simulink model "control_sim_PI_non_linear_noise"  (R2024b)
settings: Solver=ode4  StartTime=0.0  StopTime=150  FixedStep=0.001  RelTol=1e-3
libraries: simulink x1, slpidlib x1
settings Model: Creator=henri  LastModifiedBy=guilherme-lazzarini
settings ConfigComp: CovBoundaryAbsTol=1.0e-5

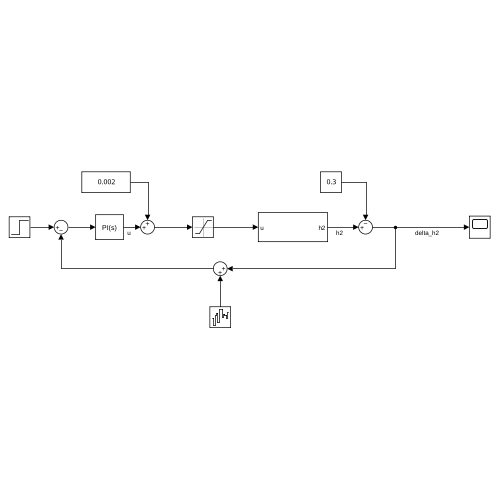
[thumbnail: Simulink's stored preview of the top-level diagram]
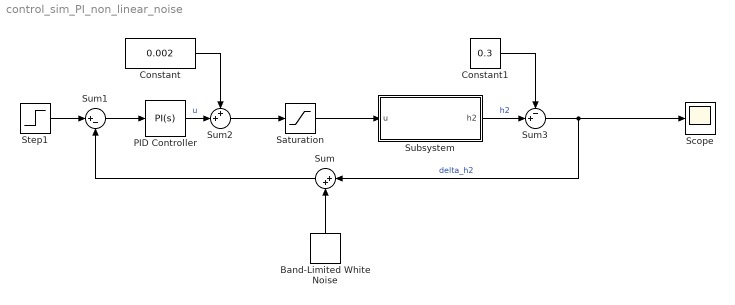
== system control_sim_PI_non_linear_noise ==
  Band-Limited White Noise : simulink/Sources/Band-Limited White Noise  Cov=[0.0001]  Ts=0.1  seed=[23341]
  Constant : Constant  Value=0.002
  Constant1 : Constant  Value=0.3
  PID Controller : slpidlib/PID Controller  Controller=PI  Form=Parallel  TimeDomain=Continuous-time  UseExternalTs=off  SampleTime=-1  IntegratorMethod=Forward Euler  FilterMethod=Forward Euler  ControllerParametersSource=internal  P=0.17  I=0.005  UseKiTs=off  D=1.75  UseExternalDerivativeSource=off  N=100  UseFilter=on  TunerSelectOption=Transfer Function Based (PID Tuner App)  InitialConditionSource=internal  InitialConditionForIntegrator=0  InitialConditionForFilter=0  DifferentiatorICPrevScaledInput=0  ExternalReset=none  TrackingMode=off  Kt=1  LimitOutput=off  SatLimitsSource=internal  UpperSaturationLimit=inf  LowerSaturationLimit=-inf  LinearizeAsGain=on  AntiWindupMode=none  Kb=1  LimitIntegrator=off  UpperIntegratorSaturationLimit=inf  LowerIntegratorSaturationLimit=-inf  POutMin=[]  POutMax=[]  IOutMin=[]  IOutMax=[]  DOutMin=[]  DOutMax=[]  NOutMin=[]  NOutMax=[]  SumOutMin=[]  SumOutMax=[]  SaturationOutMin=[]  SaturationOutMax=[]  PParamMin=[]  PParamMax=[]  IParamMin=[]  IParamMax=[]  DParamMin=[]  DParamMax=[]  NParamMin=[]  NParamMax=[]  KbParamMin=[]  KbParamMax=[]  KtParamMin=[]  KtParamMax=[]  KbOutMin=[]  KbOutMax=[]  KtOutMin=[]  KtOutMax=[]  IntegratorOutMin=[]  IntegratorOutMax=[]  FilterOutMin=[]  FilterOutMax=[]  SumI1OutMin=[]  SumI1OutMax=[]  SumI2OutMin=[]  SumI2OutMax=[]  SumI3OutMin=[]  SumI3OutMax=[]  SumI4OutMin=[]  SumI4OutMax=[]  SumDOutMin=[]  SumDOutMax=[]  DifferentiatorOutMin=[]  DifferentiatorOutMax=[]  FilterDiffOutCoefMin=[]  FilterDiffOutCoefMax=[]  ReciprocalOutMin=[]  ReciprocalOutMax=[]  SumDenOutMin=[]  SumDenOutMax=[]  SumNumOutMin=[]  SumNumOutMax=[]  DivideOutMin=[]  DivideOutMax=[]  UdiffTsProdOutMin=[]  UdiffTsProdOutMax=[]  NTsProdOutMin=[]  NTsProdOutMax=[]  UintegralTsProdOutMin=[]  UintegralTsProdOutMax=[]  UngainTsProdOutMin=[]  UngainTsProdOutMax=[]  ClampingZeroOutDataTypeStr=Inherit: Inherit via back propagation  ClampingZeroOutMin=[]  ClampingZeroOutMax=[]  FilterDenConstantOutDataTypeStr=Inherit: Inherit via back propagation  FilterDenConstantOutMin=[]  FilterDenConstantOutMax=[]  PCopyOutDataTypeStr=Inherit: Inherit via back propagation  PCopyOutMin=[]  PCopyOutMax=[]  NCopyOutDataTypeStr=Inherit: Inherit via back propagation  NCopyOutMin=[]  NCopyOutMax=[]  IntegratorContinuousStateAttributes=''  IntegratorStateMustResolveToSignalObject=off  IntegratorRTWStateStorageClass=Auto  FilterContinuousStateAttributes=''  FilterStateMustResolveToSignalObject=off  FilterRTWStateStorageClass=Auto  ParallelPVariant=InternalParameters  IdealPVariant=Disabled  IVariant=InternalParameters  DVariant=Disabled  IntegratorVariant=Continuous  SatVariant=Disabled  AWVariant=Passthrough  PCopyVariant=Disabled  TRVariant=Disabled  FdbkBlocksVariant=Forward  IdealPFdbkVariant=Disabled  SatFdbkVariant=Disabled  DerivativeFilterVariant=Disabled  NVariant=Disabled  NCopyVariant=Disabled_SignalSpec  FilterICVariant=Disabled  IntegratorICVariant=InternalICs  ExternalResetVariant=Disabled  TRSumVariant=Passthrough  SumFdbkVariant=Disabled  SumVariant=Sum_PI  TsampFilterVariant=InternalTs  TsampNgainVariant=Passthrough  TsampIntegralVariant=Disabled_SignalSpec  ExternalSaturationOutDataTypeStr=Inherit: Same as second input  DerivativeSourceVariant=Disabled  PreIntVariant=InternalPreInt
  Saturation : Saturate
  Scope : Scope
  Step1 : Step  After=0.8  SampleTime=0
  Subsystem : Subsystem
  Sum : Sum  Inputs=|++
  Sum1 : Sum  Inputs=|+-
  Sum2 : Sum  Inputs=++|
  Sum3 : Sum  Inputs=-+|
  wires:
  Sum1/1 -> PID Controller/1
  Sum3/1 -> Sum/1, Scope/1  "delta_h2"
  Constant1/1 -> Sum3/1
  Subsystem/1(h2) -> Sum3/2  "h2"
  Step1/1 -> Sum1/1
  Constant/1 -> Sum2/1
  PID Controller/1 -> Sum2/2  "u"
  Sum2/1 -> Saturation/1
  Saturation/1 -> Subsystem/1(u)
  Band-Limited White Noise/1 -> Sum/2
  Sum/1 -> Sum1/2

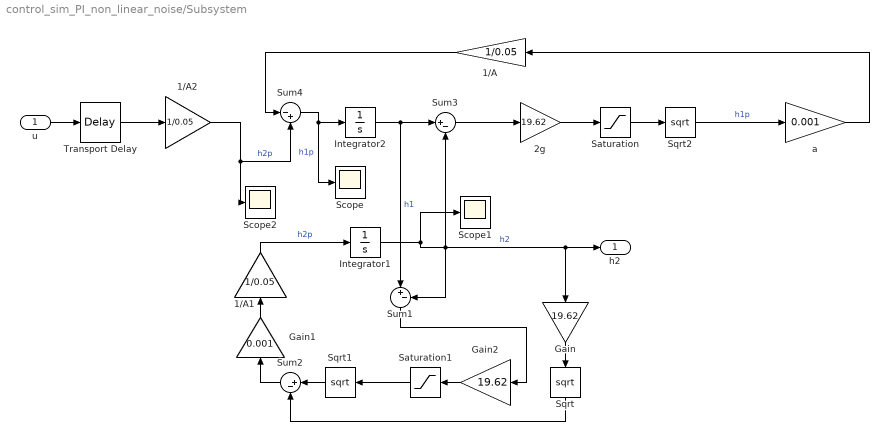
== system control_sim_PI_non_linear_noise/Subsystem ==
  u : Inport
  1/A : Gain  Gain=1/0.05
  1/A1 : Gain  Gain=1/0.05
  1/A2 : Gain  Gain=1/0.05
  2g : Gain  Gain=19.62
  Gain : Gain  Gain=19.62
  Gain1 : Gain  Gain=0.001
  Gain2 : Gain  Gain=19.62
  Integrator1 : Integrator  InitialCondition=0.3
  Integrator2 : Integrator  InitialCondition=0.6
  Saturation : Saturate  UpperLimit=inf  LowerLimit=0
  Saturation1 : Saturate  UpperLimit=inf  LowerLimit=0
  Scope : Scope
  Scope1 : Scope
  Scope2 : Scope
  Sqrt : Sqrt
  Sqrt1 : Sqrt
  Sqrt2 : Sqrt
  Sum1 : Sum  Inputs=|+-
  Sum2 : Sum  Inputs=|+-
  Sum3 : Sum  Inputs=|+-
  Sum4 : Sum  Inputs=|-+
  Transport Delay : TransportDelay  DelayTime=0.005
  a : Gain  Gain=0.001
  h2 : Outport
  wires:
  Sqrt/1 -> Sum2/2
  Sum3/1 -> 2g/1
  2g/1 -> Saturation/1
  Gain2/1 -> Saturation1/1
  Gain/1 -> Sqrt/1
  Integrator1/1 -> Sum3/2, h2/1, Gain/1, Sum1/2, Scope1/1  "h2"
  Integrator2/1 -> Sum3/1, Sum1/1  "h1"
  Sum2/1 -> Gain1/1
  Sqrt1/1 -> Sum2/1
  Sum1/1 -> Gain2/1
  u/1 -> Transport Delay/1
  a/1 -> 1/A/1
  Sum4/1 -> Scope/1, Integrator2/1  "h1p"
  1/A/1 -> Sum4/1
  1/A1/1 -> Integrator1/1  "h2p"
  Gain1/1 -> 1/A1/1
  Transport Delay/1 -> 1/A2/1
  1/A2/1 -> Scope2/1, Sum4/2  "h2p"
  Sqrt2/1 -> a/1  "h1p"
  Saturation/1 -> Sqrt2/1
  Saturation1/1 -> Sqrt1/1
